simulink library "DQsym_Lib"  (R2024a)
settings: Solver=VariableStepAuto  StartTime=0.0  StopTime=10.0  RelTol=1e-3
undefined symbols (not defined in the file or in its folder): N, S, Ts_dqn, Vnom_prim
settings Model: Creator=Robert  LastModifiedBy=salsarayreh
settings DebuggingCC: UnconnectedInputMsg=warning  UnconnectedOutputMsg=warning  UnconnectedLineMsg=warning
settings ModelReferenceCC: EnableRefExpFcnMdlSchedulingChecks=on
settings RTWCC: GPUComputeCapability=3.5  DLArmComputeVersion=19.05

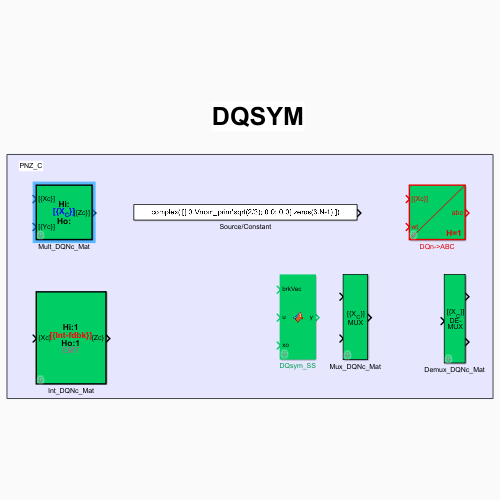
[thumbnail: Simulink's stored preview of the top-level diagram]
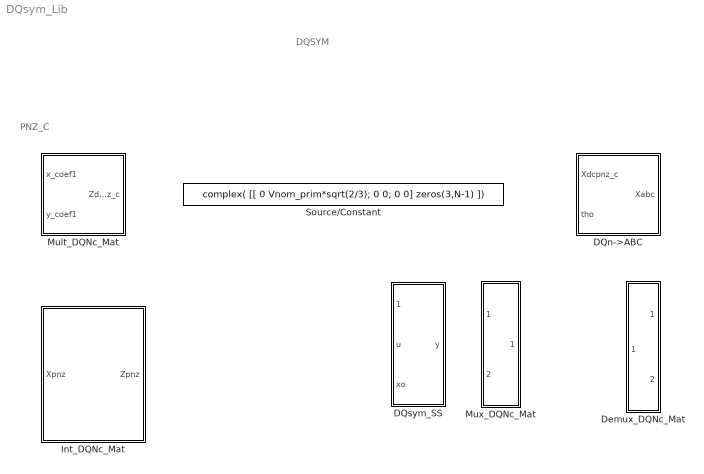
== system DQsym_Lib ==
  note: PNZ_C
  note: DQSYM
  DQn->ABC : MATLAB Function  TreatAsAtomicUnit=on  mask{N=1}
      mask prompts: N "Harmonic order:"
  DQsym_SS : MATLAB Function  TreatAsAtomicUnit=on  mask{Ad=S.A, Bd=S.B, Cd=S.C, Dd=S.D, swOnRes=1e-3*ones(1,6), swOffRes=1e6*ones(1,6), swType=ones(1,6), dt=2e-5, nrSWvec=6}
      mask prompts: Ad "A"; Bd "B"; Cd "C"; Dd "D"; swOnRes "Switch on resistance:"; swOffRes "Switch off resistance:"; swType "Switch type:"; dt "Time step (s):"; nrSWvec "Number of switches:"
  Demux_DQNc_Mat : Subsystem  mask{nrOut=2}
      mask prompts: nrOut "Number of outputs [{C}]"
      mask init:
      | if(isempty(nrOut))
      |     Simulink.SubSystem.deleteContents(gcb);
      | else
      | 
      |     IndexOptionArray = cell(2,1);
      |     IndexOptionArray(1) = {'Select all'           };
      |     IndexOptionArray(2) = {'Index vector (dialog)'};
      | 
      |     PortHandles = get_param(gcb,'PortHandles');
      | 
      |     lenOut = length(PortHandles.Outport);
      | 
      |     if(nrOut ~= lenOut) % Important to avoid reinitialization of the block!
      | 
      |         Simulink.SubSystem.deleteContents(gcb);
      | 
      |         add_block('built-in/Inport',[gcb,strcat('/In',num2str(1))]);
      |         set_param([gcb,strcat('/In',num2str(1))],'position' , [50,65+1*50,90,85+1*50]);
      | 
      |         for i = 1 : nrOut
      |             add_block('simulink/Signal Routing/Selector',[gcb,strcat('/Sel',num2str(i))],...
      |                 'IndexOptionArray',IndexOptionArray,...
      |                 'NumberOfDimensions','2',...
      |                 'IndexOptions','Index vector (dialog),Select all',...
      |                 'Indices',strcat(num2str((i-1)*3+1),':',num2str((i-1)*3+3),', 1') ...
      |                 );
      |             set_param([gcb,strcat('/Sel',num2str(i))],'position' , [450,65+i*50,490,85+i*50])
      | 
      | 
      |             add_block('built-in/Outport',[gcb,strcat('/Out',num2str(i))]);
      |             set_param([gcb,strcat('/Out',num2str(i))],'position' , [750,65+i*50,790,85+i*50]);
      | 
      |             add_line(gcb,strcat('In',num2str(1),'/1'),  strcat('Sel',num2str(i),'/1'),'autorouting','on');
      |             add_line(gcb,strcat('Sel',num2str(i),'/1'), strcat('Out',num2str(i),'/1'),'autorouting','on');
      |         end
      | 
      |     end
      | 
      | end
      mask Display: disp(['{\color{red}\bf\fontsize{12}} [\{X_C\}]',newline,' DE-',newline,' MUX'], 'texmode','on');
  Int_DQNc_Mat : MATLAB Function  TreatAsAtomicUnit=on  mask{N=1, dt=50e-6, w=2*pi*50, InitInt=zeros(3,1), swFeed=on, R=eye(3), iL=eye(3)}
      mask prompts: N "Order number:"; dt "Time step (s):"; w "Angular frequency (1/rad):"; InitInt "Initial conditions DC [3x1]:"; swFeed "Enable feedback"; R "Feedback parameter (Kr {abc}):"; iL "Feedback parameter (Ki {abc}):"
  Mult_DQNc_Mat : MATLAB Function  TreatAsAtomicUnit=on  SystemSampleTime=Ts_dqn  mask{N=N, HrmDbl=on}
      mask prompts: N "Harmonic order:"; HrmDbl "Double Harmonic"
  Mux_DQNc_Mat : Subsystem  mask{nrInp=2}
      mask prompts: nrInp "Number of inputs [{C}]"
      mask init:
      | %blocks = find_system(gcb,'LookUnderMasks','on','FollowLinks','on')
      | %set_param(gcb, 'MaskSelfModifiable', 'on');
      | 
      | % if(SSM == [])
      | %     Simulink.SubSystem.deleteContents(gcb);
      | % else
      | 
      | if(isempty(nrInp))
      |     Simulink.SubSystem.deleteContents(gcb);
      | else
      | 
      |     nrOut = 1;
      | 
      | 
      | PortHandles = get_param(gcb,'PortHandles');
      | lenInp = length(PortHandles.Inport);
      | lenOut = length(PortHandles.Inport);
      | 
      | if(nrInp ~= lenInp)
      |     %disp('ENTERED')
      |     Simulink.SubSystem.deleteContents(gcb);
      | %     add_block('simulink/Continuous/State-Space', [gcb,'/ss_block'], 'A','SS.A', 'B','SS.B', 'C','SS.C', 'D','SS.D', 'X0','X0')
      | %     set_param([gcb,'/ss_block'],'position' , [350,100,450,150])
      | 
      | 
      | 
      |         add_block('simulink/Math Operations/Matrix Concatenate',[gcb,'/Mux'], 'NumInputs',num2str(nrInp), 'ConcatenateDimension',num2str(1));
      |         set_param([gcb,'/Mux'],'position' , [200,100,250,100+nrInp*50])
      |         
      | %         add_block('built-in/Demux',[gcb,'/Demux'], 'Outputs',num2str(nrOut));
      | %         set_param([gcb,'/Demux'],'position' , [500,100,550,100+nrOut*50])
      | 
      | 
      |         for i = 1 : nrInp
      |             add_block('built-in/Inport',[gcb,strcat('/In',num2str(i))]);
      |             set_param([gcb,strcat('/In',num2str(i))],'position' , [50,65+i*50,90,85+i*50]);
      |             add_line(gcb,strcat('In',num2str(i),'/1'),strcat('Mux/',num2str(i)),'autorouting','on');
      |         end
      | 
      |         for i = 1 : nrOut
      |             add_block('built-in/Outport',[gcb,strcat('/Out',num2str(i))]);
      |             set_param([gcb,strcat('/Out',num2str(i))],'position' , [750,65+i*50,790,85+i*50]);
      |             add_line(gcb,strcat('Mux/',num2str(i)), strcat('Out',num2str(i),'/1'),'autorouting','on');
      |         end
      | 
      | 
      | %     add_line(gcb, 'Mux/1', 'ss_block/1')
      | %     add_line(gcb, 'ss_block/1', 'Demux/1')
      | 
      | end
      | 
      | end
      mask Display: disp(['{\color{red}\bf\fontsize{12}} [\{X_C\}]',newline,' MUX'], 'texmode','on');
  Source/Constant : Constant  Value=complex( [[ 0 Vnom_prim*sqrt(2/3); 0 0; 0 0] zeros(3,N-1) ])

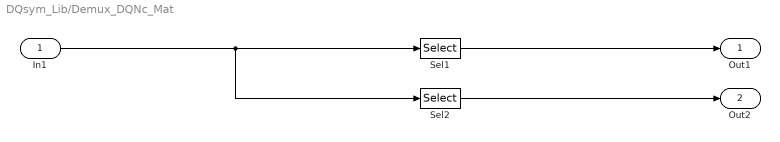
== system DQsym_Lib/Demux_DQNc_Mat ==
  In1 : Inport
  Sel1 : Selector  NumberOfDimensions=2  InputPortWidth=3  IndexOptions=Index vector (dialog),Select all  Indices=1:3, 1  OutputSizes=1
  Sel2 : Selector  NumberOfDimensions=2  InputPortWidth=3  IndexOptions=Index vector (dialog),Select all  Indices=4:6, 1  OutputSizes=1
  Out1 : Outport
  Out2 : Outport  Port=2
  wires:
  In1/1 -> Sel1/1, Sel2/1
  Sel1/1 -> Out1/1
  Sel2/1 -> Out2/1

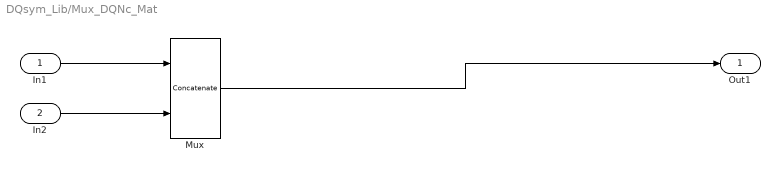
== system DQsym_Lib/Mux_DQNc_Mat ==
  In1 : Inport
  In2 : Inport  Port=2
  Mux : Concatenate  Mode=Multidimensional array  ConcatenateDimension=nrOut
  Out1 : Outport
  wires:
  In1/1 -> Mux/1
  In2/1 -> Mux/2
  Mux/1 -> Out1/1

== matlab function DQsym_Lib/Mult_DQNc_Mat ==
  data: x_coef1 input; y_coef1 input; N parameter; Zdcpnz_c output
function Zdcpnz_c = SICO_DPs_3ph(x_coef1, y_coef1, N) %#codegen

MAX_N = 10;
MAX_L = MAX_N + 1;
MAX_K = 2*MAX_N;

assert(N >= 0 && N <= MAX_N);

persistent Sas Ssa
if isempty(Sas)
    a  = complex(-0.5,  0.8660254037844386);
    a2 = complex(-0.5, -0.8660254037844386);
    Sas = [1, a, a2;
           1, a2, a;
           1, 1, 1] / 3;
    Ssa = inv(Sas);
end

L = N + 1;
max_k = 2*N;

% Always fixed-size output
Zdcpnz_c = complex(zeros(3, 2*MAX_N+1));

x_coef2 = complex(zeros(3, MAX_L));
y_coef2 = complex(zeros(3, MAX_L));

nx = min(size(x_coef1,2), L);
ny = min(size(y_coef1,2), L);

x_coef2(:,1:nx) = x_coef1(:,1:nx);
y_coef2(:,1:ny) = y_coef1(:,1:ny);

x_coef3 = Ssa * x_coef2;
y_coef3 = Ssa * y_coef2;

xy_phasors = complex(zeros(3, MAX_K+1));
Cs = zeros(3, MAX_K+1);
Cc = zeros(3, MAX_K+1);
C0 = zeros(3,1);

for m = 0:N
    axs = real(x_coef3(:,m+1));
    axc = imag(x_coef3(:,m+1));

    for n = 0:N
        bxs = real(y_coef3(:,n+1));
        bxc = imag(y_coef3(:,n+1));

        if m == 0 && n == 0
            C0 = C0 + real(x_coef3(:,1)) .* real(y_coef3(:,1));
        end

        if m == n && m > 0
            C0 = C0 + 0.5*axs.*bxs + 0.5*axc.*bxc;
        end

        if m > 0 && n > 0
            k_plus  = m + n;
            k_minus = abs(m - n);
            s = sign(m - n);

            Cs(:,k_plus+1) = Cs(:,k_plus+1) + 0.5*axs.*bxc + 0.5*axc.*bxs;
            Cc(:,k_plus+1) = Cc(:,k_plus+1) + 0.5*axc.*bxc - 0.5*axs.*bxs;

            if k_minus > 0
                Cs(:,k_minus+1) = Cs(:,k_minus+1) + 0.5*s*axs.*bxc - 0.5*s*axc.*bxs;
                Cc(:,k_minus+1) = Cc(:,k_minus+1) + 0.5*axc.*bxc + 0.5*axs.*bxs;
            end
        end

        if m == 0 && n > 0
            Cs(:,n+1) = Cs(:,n+1) + real(x_coef3(:,1)).*bxs;
            Cc(:,n+1) = Cc(:,n+1) + real(x_coef3(:,1)).*bxc;
        end

        if n == 0 && m > 0
            Cs(:,m+1) = Cs(:,m+1) + real(y_coef3(:,1)).*axs;
            Cc(:,m+1) = Cc(:,m+1) + real(y_coef3(:,1)).*axc;
        end
    end
end

xy_phasors(:,1) = complex(C0,0);
for k = 1:max_k
    xy_phasors(:,k+1) = complex(Cs(:,k+1), Cc(:,k+1));
end

tmp = Sas * xy_phasors(:,1:max_k+1);
Zdcpnz_c(:,1:max_k+1) = tmp;

== matlab function DQsym_Lib/DQn->ABC ==
  data: Xdcpnz_c input; tho input; Xabc output; N parameter
%function abc = Mult(Z0,Zdp,Zqp,Zdn,Zqn,Zdz,Zqz,th, N)
function Xabc = dqn2abc(Xdcpnz_c,tho,N)

    persistent Sas;
    persistent Ssa;

    if(isempty(Sas)) 
        a = -0.5+0.866i;
        a2 = -0.5-0.866i;
        Sas = [1,a,a2;1,a2,a;1,1,1]/3;
        Ssa = eye(3)/(Sas);
    end

    Xabc = zeros(3,1);

    for i = 1 : N+1
    
    
        if(i>1)
            h = i-1;
    
            th = h*tho;
        
            mag_p = abs(Xdcpnz_c(1,i));
            ang_p = angle(Xdcpnz_c(1,i));
            mag_n = abs(Xdcpnz_c(2,i));
            ang_n = angle(Xdcpnz_c(2,i));
            mag_z = abs(Xdcpnz_c(3,i));
            ang_z = angle(Xdcpnz_c(3,i));
            
            abc3p = mag_p*[sin(th+ang_p) ; sin(th+ang_p-2*pi/3) ; sin(th+ang_p+2*pi/3) ];
            abc3n = mag_n*[sin(th+ang_n) ; sin(th+ang_n+2*pi/3) ; sin(th+ang_n-2*pi/3) ];
            abc3z = mag_z*[sin(th+ang_z) ; sin(th+ang_z)        ; sin(th+ang_z)  ];
        
            Xabc = Xabc + abc3p+abc3n+abc3z;
        else
            Xabc = Xabc + real(Ssa*(Xdcpnz_c(:,1)));
        
        end
    
        
    end

end

== matlab function DQsym_Lib/Int_DQNc_Mat ==
  settings: updateMethod=DISCRETE
  data: Xpnz input; N parameter; dt parameter; w parameter; InitInt parameter; Zpnz output; R parameter; iL parameter; swFeed parameter
function Zpnz    = Int_DQN_Mat(Xpnz, N, dt, w, InitInt, R, iL, swFeed)


    nrSig = size(Xpnz,1)/3;
    Zpnz = complex(zeros(nrSig*3,N+1));

    persistent Zpnz_old;
    persistent Xpnz_old;
    persistent Krl1;
    persistent Krl2;
    persistent dt2;
        
    if(isempty(Zpnz_old)) 
    


        
        % if(~isempty(InitInt))
        % Zpnz_old(:,1) = Sas * InitInt;
        % end


        Zpnz_old = complex(zeros(nrSig*3,N+1));
        Xpnz_old = complex(zeros(nrSig*3,N+1));
        dt2 = dt/2;

        if(swFeed)
            mrows = size(R,1)/3; %signal size
            mcols = size(R,2)/3; %signal size

            szMatR = size(R,1);
            szMatiL = size(iL,1);

            if(szMatiL ~= szMatR || size(R,1) ~= size(R,2) || size(iL,1) ~= size(iL,2))
                error('[Int_DQN_Mat/swFeedback] check matrix sizes!');
            end
    
            Rpnz = complex(zeros(3*mrows,3*mcols));
            iLpnz = complex(zeros(3*mrows,3*mcols));

            a = -0.5+0.866i;
            a2 = -0.5-0.866i;
            Sas = [1,a,a2;1,a2,a;1,1,1]/3;
    
            for i = 1 : mrows
                for j = 1 : mcols
                     Rpnz((1:3) + (i-1)*3,(1:3) + (j-1)*3) = Sas*R((1:3) + (i-1)*3,(1:3) + (j-1)*3)/Sas;
                    iLpnz((1:3) + (i-1)*3,(1:3) + (j-1)*3) = Sas*iL((1:3) + (i-1)*3,(1:3) + (j-1)*3)/Sas;
                end
            end

            Rpnz  = diag(diag(real(Rpnz)));
            iLpnz = diag(diag(real(iLpnz)));

            Krl1 = (iLpnz/(eye(szMatR)+dt2*Rpnz*iLpnz));
            Krl2 = (eye(szMatR)-dt2*Rpnz*iLpnz)/(eye(szMatR)+dt2*Rpnz*iLpnz);
        else
            Krl1 = 1;
            Krl2 = 1;
        end
            
    end

    if(swFeed)
        Zpnz(:,1) = Krl1*dt2*(Xpnz(:,1)+Xpnz_old(:,1))+Krl2*Zpnz_old(:,1);
    else
        Zpnz(:,1) = dt2*(Xpnz(:,1)+Xpnz_old(:,1))+Zpnz_old(:,1);
    end

    Xpnz_old(:,1) = Xpnz(:,1);
    Zpnz_old(:,1) = Zpnz(:,1);

    for i = 1 : N
        if(N>0)
            wn =  i * w; 
            wndt2 = wn*dt2;

            A = 2*dt2/(1+wndt2^2);
            B = (1-wndt2^2)/(1+wndt2^2);

            if(swFeed)

                Zpnz(:,i+1) =      Krl1*A*(real(Xpnz(:,i+1))+wndt2*imag(Xpnz(:,i+1)))+Krl2*(B*real(Zpnz_old(:,i+1))+A*wn*imag(Zpnz_old(:,i+1))) ...
                             + 1i*(Krl1*A*(imag(Xpnz(:,i+1))-wndt2*real(Xpnz(:,i+1)))+Krl2*(B*imag(Zpnz_old(:,i+1))-A*wn*real(Zpnz_old(:,i+1))));
            else
                Zpnz(:,i+1) =      A*(real(Xpnz(:,i+1))+wndt2*imag(Xpnz(:,i+1)))+(B*real(Zpnz_old(:,i+1))+A*wn*imag(Zpnz_old(:,i+1))) ...
                             + 1i*(A*(imag(Xpnz(:,i+1))-wndt2*real(Xpnz(:,i+1)))+(B*imag(Zpnz_old(:,i+1))-A*wn*real(Zpnz_old(:,i+1))));
            end

            Zpnz_old(:,i+1) = Zpnz(:,i+1);

        end
    end


end

== matlab function DQsym_Lib/DQsym_SS ==
  data: Ad parameter; Bd parameter; Cd parameter; Dd parameter; swOnRes parameter; swOffRes parameter; swType parameter; brkVec input; y output [1..100]; u input; xo input
function y  = nFdss2(Ad, Bd, Cd, Dd, swOnRes, swOffRes, swType, brkVec, u,xo)

% INIT


persistent Ads;
persistent Bds;
persistent Cds;
persistent Dds;
persistent x;
persistent x_old;
persistent swVec;
persistent swVecOld;
persistent nSwitches;
persistent nStates;
persistent nOutputs;
persistent nInputs;
persistent yswitch;
persistent xkm12;   % First half-step state at t - Ts/2
persistent xkp12;   % Second half-step state at t + Ts/2
persistent xCorrected; % Corrected state at time t


x = complex(zeros(size(Ad,1),size(u,2)));
y = complex(zeros(size(Cd,1),size(u,2)));


% Adc= Ad; Bdc = Bd ; Cdc = Cd; Ddc = Dd;

[Adc, Bdc, Cdc, Ddc] = convertToPhasor(Ad, Bd, Cd, Dd);
% Initialization (First Call)

if isempty(x_old)

    if (swType ~= 0)
    
        nStates = size(Ad, 1);
        nInputs = size(Bd, 2);
        nOutputs = size(Cd, 1);
        nSwitches = sum(swType == 1);

        x_old = complex([xo,zeros(size(xo,1),size(u,2)-1)]);
        xCorrected = x_old;

        swVec = brkVec;
        swVecOld = swVec;

        yswitch = complex(zeros(nSwitches));


        xkp12 = complex(zeros(nStates, 1));
        xkm12 = complex(zeros(nStates, 1));

         % First Half-step Correction: xkm12 at t - Ts/2 % Before Updating Matrices

            % Calculate using old state (x_old) and unmodified matrices (Ads, Bds)
            for j = 1:nStates
                for i = 1:nStates
                    if i == j
                        xkm12(i) = xkm12(i) + (Adc(i, j) + 1) * 0.5 * x_old(j);
                    else
                        xkm12(i) = xkm12(i) + Adc(i, j) * 0.5 * x_old(j);
                    end
                end
            end

            % Matrix B Contribution for First Half-step
            for j = 1:nInputs
                for i = 1:nStates
                    xkm12(i) = xkm12(i) + Bdc(i, j) * 0.5 * u(j);
                end
            end


    
        % Detect switch changes
        SwitchChange = (swVecOld ~= swVec);
        idxSwChng = find(SwitchChange == 1); % Indices of changed switches
        nbSwChng = sum(SwitchChange == 1);   % Number of switches that changed

        % Update switching conductance
        for s = 1:nSwitches
            if swVec(s) == 1
                yswitch(s) = complex(1 / swOnRes(s));
            else
                yswitch(s) = complex(1 / swOffRes(s));
            end
        end

        % Initialize DxCol and BDcol (for matrix updates)
        DxCol = complex(zeros(nOutputs, 1));
        BDcol = complex(zeros(nStates, 1));

        % Process each switch change
        for k = 1:nbSwChng
            nSw = idxSwChng(k);  % Get switch index
            kSw = SwitchChange(nSw);  % Get new switch state

            % Compute DxCol update for D matrix
            tmp = Ddc(nSw, nSw) * yswitch(nSw);
            temp = complex(1 / (1 - tmp * kSw));
            temp2 = yswitch(nSw) * temp * kSw;

            for i = 1:nOutputs
                DxCol(i) = Ddc(i, nSw) * temp2;
            end
            DxCol(nSw) = temp;

            % Compute BDcol update for B matrix
            temp2 = yswitch(nSw) * kSw;
            for i = 1:nStates
                BDcol(i) = Bdc(i, nSw) * temp2;
            end

            % Copy row nSw of Cd and zero it out
            tmp1 = Cdc(nSw, :);
            Cdc(nSw, :) = complex(0);

            % Copy row nSw of Dd and zero it out
            tmp2 = Ddc(nSw, :);
            Ddc(nSw, :) = complex(0);

            % Update C and D matrices
            for i = 1:nOutputs
                for j = 1:nStates
                    Cdc(i, j) = Cdc(i, j) + DxCol(i) * tmp1(j);
                end
                for j = 1:nInputs
                    Ddc(i, j) = Ddc(i, j) + DxCol(i) * tmp2(j);
                end
            end

            % Update A and B matrices
            for i = 1:nStates
                for j = 1:nStates
                    Adc(i, j) = Adc(i, j) + BDcol(i) * Cdc(nSw, j);
                end
                for j = 1:nInputs
                    Bdc(i, j) = Bdc(i, j) + BDcol(i) * Ddc(nSw, j);
                end
            end
        end


        % Store updated matrices
        Ads = Adc;
        Bds = Bdc;
        Cds = Cdc;
        Dds = Ddc;

           % SECOND HALF-STEP CORRECTION % After Updating Matrices


            for j = 1:nStates
                for i = 1:nStates
                    if i == j
                        xkp12(i) = xkp12(i) + (Ads(i, j) + 1) * 0.5 * x_old(j);
                    else
                        xkp12(i) = xkp12(i) + Ads(i, j) * 0.5 * x_old(j);
                    end
                end
            end

            % Matrix B Contribution for Second Half-step
            for j = 1:nInputs
                for i = 1:nStates
                    xkp12(i) = xkp12(i) + Bds(i, j) * 0.5 * u(j);
                end
            end


    % Store old switch vector for next iteration
        swVecOld = swVec;

        x_old(:,1) = (xkp12 + xkm12) * 0.5;

     else
        nStates = size(Ad, 1);
        nInputs = size(Bd, 2);
        nOutputs = size(Cd, 1);
        nSwitches = sum(swType == 1);

        x_old = complex([xo,zeros(size(xo,1),size(u,2)-1)]);
        xCorrected = x_old;

        swVec = brkVec;
        swVecOld = swVec;

        Ads = Adc;
        Bds = Bdc;
        Cds = Cdc;
        Dds = Ddc;
    end
end

% Update switch vector
if (swType ~= 0)
    swVec = brkVec;
end


% DETECT SWITCH CHANGES AND UPDATE MATRICES

if (any(swType ~= 0) && any(swVecOld ~= swVec))

        nStates = size(Ad, 1);
        nInputs = size(Bd, 2);
        nOutputs = size(Cd, 1);
        nSwitches = sum(swType == 1);
        
        yswitch = complex(zeros(nSwitches));

        xkp12 = complex(zeros(nStates, 1));
        xkm12 = complex(zeros(nStates, 1));

        % First Half-step Correction: xkm12 at t - Ts/2 % Before Updating Matrices

            % Calculate using old state (x_old) and unmodified matrices (Ads, Bds)
            for j = 1:nStates
                for i = 1:nStates
                    if i == j
                        xkm12(i) = xkm12(i) + (Ads(i, j) + 1) * 0.5 * x_old(j);
                    else
                        xkm12(i) = xkm12(i) + Ads(i, j) * 0.5 * x_old(j);
                    end
                end
            end

            % Matrix B Contribution for First Half-step
            for j = 1:nInputs
                for i = 1:nStates
                    xkm12(i) = xkm12(i) + Bds(i, j) * 0.5 * u(j);
                end
            end



       % Detect switch changes
        SwitchChange = (swVecOld ~= swVec);
        idxSwChng = find(SwitchChange == 1); % Indices of changed switches
        nbSwChng = sum(SwitchChange == 1);   % Number of switches that changed

        % Update switching conductance
        for s = 1:nSwitches
            if swVec(s) == 1
                yswitch(s) = complex(1 / swOnRes(s));
            else
                yswitch(s) = complex(1 / swOffRes(s));
            end
        end

        % Initialize DxCol and BDcol (for matrix updates)
        DxCol = complex(zeros(nOutputs, 1));
        BDcol = complex(zeros(nStates, 1));

        % Process each switch change
        for k = 1:nbSwChng
            nSw = idxSwChng(k);  % Get switch index
            kSw = SwitchChange(nSw);  % Get new switch state

            % Compute DxCol update for D matrix
            tmp = Dds(nSw, nSw) * yswitch(nSw);
            temp = complex(1 / (1 - tmp * kSw));
            temp2 = yswitch(nSw) * temp * kSw;

            for i = 1:nOutputs
                DxCol(i) = Dds(i, nSw) * temp2;
            end
            DxCol(nSw) = temp;

            % Compute BDcol update for B matrix
            temp2 = yswitch(nSw) * kSw;
            for i = 1:nStates
                BDcol(i) = Bds(i, nSw) * temp2;
            end

            % Copy row nSw of Cd and zero it out
            tmp1 = Cds(nSw, :);
            Cds(nSw, :) = complex(0);

            % Copy row nSw of Dd and zero it out
            tmp2 = Dds(nSw, :);
            Dds(nSw, :) = complex(0);

            % Update C and D matrices
            for i = 1:nOutputs
                for j = 1:nStates
                    Cds(i, j) = Cds(i, j) + DxCol(i) * tmp1(j);
                end
                for j = 1:nInputs
                    Dds(i, j) = Dds(i, j) + DxCol(i) * tmp2(j);
                end
            end

            % Update A and B matrices
            for i = 1:nStates
                for j = 1:nStates
                    Ads(i, j) = Ads(i, j) + BDcol(i) * Cds(nSw, j);
                end
                for j = 1:nInputs
                    Bds(i, j) = Bds(i, j) + BDcol(i) * Dds(nSw, j);
                end
            end
        end


        % Store updated matrices
        % Ads;
        % Bds;
        % Cds;
        % Dds;

            
        % SECOND HALF-STEP CORRECTION % After Updating Matrices


            for j = 1:nStates
                for i = 1:nStates
                    if i == j
                        xkp12(i) = xkp12(i) + (Ads(i, j) + 1) * 0.5 * x_old(j);
                    else
                        xkp12(i) = xkp12(i) + Ads(i, j) * 0.5 * x_old(j);
                    end
                end
            end

            % Matrix B Contribution for Second Half-step
            for j = 1:nInputs
                for i = 1:nStates
                    xkp12(i) = xkp12(i) + Bds(i, j) * 0.5 * u(j);
                end
            end

    % Store old switch vector for next iteration
        swVecOld = swVec;

         x_old(:,1) = (xkp12 + xkm12) * 0.5;

end 
   
       % Ao=Ads;
       % Bo=Bds;
       % Co=Cds;
       % Do=Dds;


% STATE AND OUTPUT CALCULATION
x = Ads * x_old + Bds * u;

 x2= x *  diag(exp(-[0:(size(u,2)-1)].*2*pi*50*2e-5*1i));

x_old= x2;

% xout=xCorrected;

y = Cds * x2 + Dds * u;

end


function [Adc1, Bdc1, Cdc1, Ddc1] = convertToPhasor(A, B, C, D)

    dt= 2e-5;

    % Step 1: Discretize the matrices
    I = eye(size(A, 1));
    Ad1 = inv(I - (dt * A / 2)) * (I + (dt * A / 2));
    Bd1 = inv(I - (dt * A / 2)) * B * sqrt(dt);
    Cd1 = sqrt(dt) * C * inv(I - (dt * A / 2));
    Dd1 = D + C * inv(I - (dt * A / 2)) * (B * dt / 2);

    % 
    % Ad2= Ad1; Bd2 = Bd1; Cd2 = Cd1 ; Dd2= Dd1; 
    Ad2= A; Bd2 = B; Cd2 = C ; Dd2= D; %%temp for testing without TBE dis

    %Convert to DQN
    a = -0.5 + 0.866i;
    a2 = -0.5 - 0.866i;
    Sas = [1, a, a2; 1, a2, a; 1, 1, 1] / 3;

    % Perform the phasor transformation for each matrix
    Adc1 = transformMatrix(Ad2, Sas);
    Bdc1 = transformMatrix(Bd2, Sas);
    Cdc1 = transformMatrix(Cd2, Sas);
    Ddc1 = transformMatrix(Dd2, Sas);

end

function Mdc = transformMatrix(Md1, Sas)
    [rows, cols] = size(Md1);
    rows = rows / 3;
    cols = cols / 3;
    Mdc = complex(zeros(3 * rows, 3 * cols));
    for i = 1:rows
        for j = 1:cols
            Mdc((1:3) + (i - 1) * 3, (1:3) + (j - 1) * 3) = ...
                Sas * Md1((1:3) + (i - 1) * 3, (1:3) + (j - 1) * 3) / Sas;
        end
    end
end
